simulink model "maglev"  (R2020a)
settings: Solver=VariableStepAuto  StartTime=0.0  StopTime=10.0  RelTol=1e-3
settings Model: Creator=TomJa  LastModifiedBy=TomJa

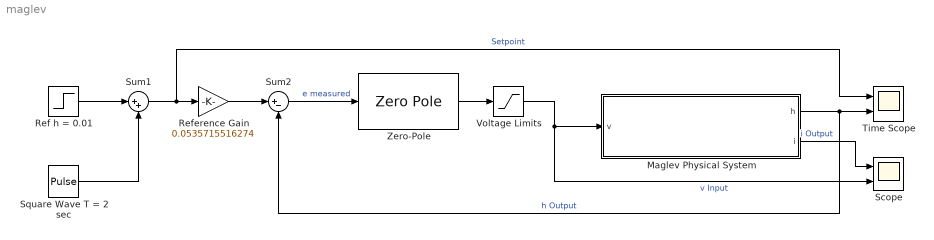
== system maglev ==
  Maglev Physical System : Subsystem
  Ref h = 0.01 : Step  Time=0  After=0.01  SampleTime=0
  Reference Gain : Gain  Gain=0.0535715516274
  Scope : Scope  NumInputPorts=2
  Square Wave T = 2 sec : DiscretePulseGenerator  PulseType=Time based  Amplitude=0.01  PulseWidth=50
  Sum1 : Sum  Inputs=|++
  Sum2 : Sum  Inputs=|+-
  Time Scope : Scope  NumInputPorts=2
  Voltage Limits : Saturate  UpperLimit=9  LowerLimit=-9
  Zero-Pole : ZeroPole  Zeros=-25  Poles=-250  Gain=-740
  wires:
  Zero-Pole/1 -> Voltage Limits/1
  Sum2/1 -> Zero-Pole/1  "e measured"
  Reference Gain/1 -> Sum2/1
  Voltage Limits/1 -> Scope/2, Maglev Physical System/1(v)  "v Input"
  Maglev Physical System/1(h) -> Time Scope/2, Sum2/2  "h Output"
  Maglev Physical System/2(i) -> Scope/1  "i Output"
  Ref h = 0.01/1 -> Sum1/1
  Sum1/1 -> Time Scope/1, Reference Gain/1  "Setpoint"
  Square Wave T = 2 sec/1 -> Sum1/2

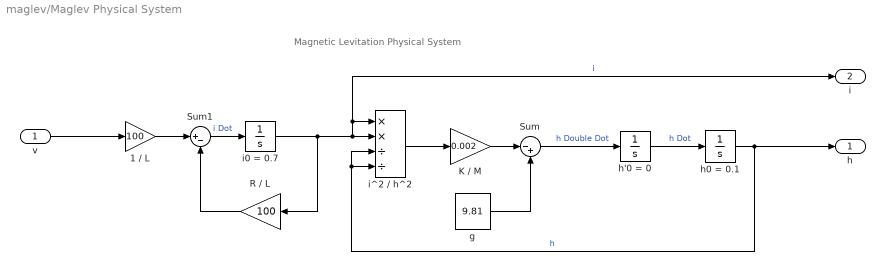
== system maglev/Maglev Physical System ==
  note: Magnetic Levitation Physical System
  v : Inport
  1 / L : Gain  Gain=100
  K / M : Gain  Gain=0.002
  R / L : Gain  Gain=100
  Sum : Sum  Inputs=|-+
  Sum1 : Sum  Inputs=|+-
  g : Constant  Value=9.81
  h'0 = 0 : Integrator
  h0 = 0.1 : Integrator  InitialCondition=.1  LimitOutput=on  UpperSaturationLimit=100  LowerSaturationLimit=0.0000000001
  i0 = 0.7 : Integrator  InitialCondition=0.700357
  i^2 / h^2 : Product  Inputs=**//
  h : Outport
  i : Outport  Port=2
  wires:
  h'0 = 0/1 -> h0 = 0.1/1  "h Dot"
  Sum1/1 -> i0 = 0.7/1  "i Dot"
  R / L/1 -> Sum1/2
  h0 = 0.1/1 -> h/1, i^2 / h^2/4, i^2 / h^2/3  "h"
  i0 = 0.7/1 -> R / L/1, i/1, i^2 / h^2/1, i^2 / h^2/2  "i"
  1 / L/1 -> Sum1/1
  Sum/1 -> h'0 = 0/1  "h Double Dot"
  K / M/1 -> Sum/1
  i^2 / h^2/1 -> K / M/1
  g/1 -> Sum/2
  v/1 -> 1 / L/1
